simulink model "REDCS_Pipeline_IntermediateModel_FSU_29APR2022"  (R2022a)
settings: Solver=VariableStepAuto  StartTime=0.0  StopTime=3600  RelTol=1e-3
values from neighbouring files (symbols this model uses):
  Ac = (pi/4)*0.6096^2    (= 0.29186350796)    [REDCS_IntermediateModel_Parameters_29APR2022.m]
  B1 = 45    [REDCS_IntermediateModel_Parameters_29APR2022.m]
  CLOSED = 0    [REDCS_IntermediateModel_Parameters_29APR2022.m]
  EP020 = 21.9    [REDCS_IntermediateModel_Parameters_29APR2022.m]
  EP022 = 13.1    [REDCS_IntermediateModel_Parameters_29APR2022.m]
  EP024 = 54.2    [REDCS_IntermediateModel_Parameters_29APR2022.m]
  EP026 = 13.4    [REDCS_IntermediateModel_Parameters_29APR2022.m]
  EP028 = 0.5    [REDCS_IntermediateModel_Parameters_29APR2022.m]
  gamma = 1.2    [REDCS_IntermediateModel_Parameters_29APR2022.m]
  J = 5    [REDCS_IntermediateModel_Parameters_29APR2022.m]
  kf = 0.05    [REDCS_IntermediateModel_Parameters_29APR2022.m]
  Lc = 20    [REDCS_IntermediateModel_Parameters_29APR2022.m]
  OPEN = 1    [REDCS_IntermediateModel_Parameters_29APR2022.m]
  r1 = 0.05    [REDCS_IntermediateModel_Parameters_29APR2022.m]
  r2 = 0.325    [REDCS_IntermediateModel_Parameters_29APR2022.m]
  sigma = 0.90    (= 0.9)    [REDCS_IntermediateModel_Parameters_29APR2022.m]
  ValveThresh = 0.001    [REDCS_IntermediateModel_Parameters_29APR2022.m]
  ZR2000 = OPEN    (= 1)    [REDCS_IntermediateModel_Parameters_29APR2022.m]
  ZR2110 = CLOSED    (= 0)    [REDCS_IntermediateModel_Parameters_29APR2022.m]
  ZR2400 = OPEN    (= 1)    [REDCS_IntermediateModel_Parameters_29APR2022.m]
  ZR2401 = 100*OPEN    (= 100)    [REDCS_IntermediateModel_Parameters_29APR2022.m]
  ZR2510 = CLOSED    (= 0)    [REDCS_IntermediateModel_Parameters_29APR2022.m]
  ZR2600 = OPEN    (= 1)    [REDCS_IntermediateModel_Parameters_29APR2022.m]
  ZR2601 = 100*OPEN    (= 100)    [REDCS_IntermediateModel_Parameters_29APR2022.m]
  ZR2700 = OPEN    (= 1)    [REDCS_IntermediateModel_Parameters_29APR2022.m]
  ZR2701 = 100*OPEN    (= 100)    [REDCS_IntermediateModel_Parameters_29APR2022.m]
  ZR2800 = OPEN    (= 1)    [REDCS_IntermediateModel_Parameters_29APR2022.m]
  ZR2801 = 100*OPEN    (= 100)    [REDCS_IntermediateModel_Parameters_29APR2022.m]
  ZR2900 = OPEN    (= 1)    [REDCS_IntermediateModel_Parameters_29APR2022.m]
  ZR2901 = 100*OPEN    (= 100)    [REDCS_IntermediateModel_Parameters_29APR2022.m]
  ZR3900 = OPEN    (= 1)    [REDCS_IntermediateModel_Parameters_29APR2022.m]
  ZR4500 = OPEN    (= 1)    [REDCS_IntermediateModel_Parameters_29APR2022.m]
  ZR5600 = OPEN    (= 1)    [REDCS_IntermediateModel_Parameters_29APR2022.m]
  ZR7800 = CLOSED    (= 0)    [REDCS_IntermediateModel_Parameters_29APR2022.m]
undefined symbols (not defined in the file or in its folder): cotd, LEG_DEMAND_10A, LEG_DEMAND_3A, magnitude
libraries: fl_lib x170, nesl_utility x109, simulink x12, slpidlib x4
(part 4 of 4)

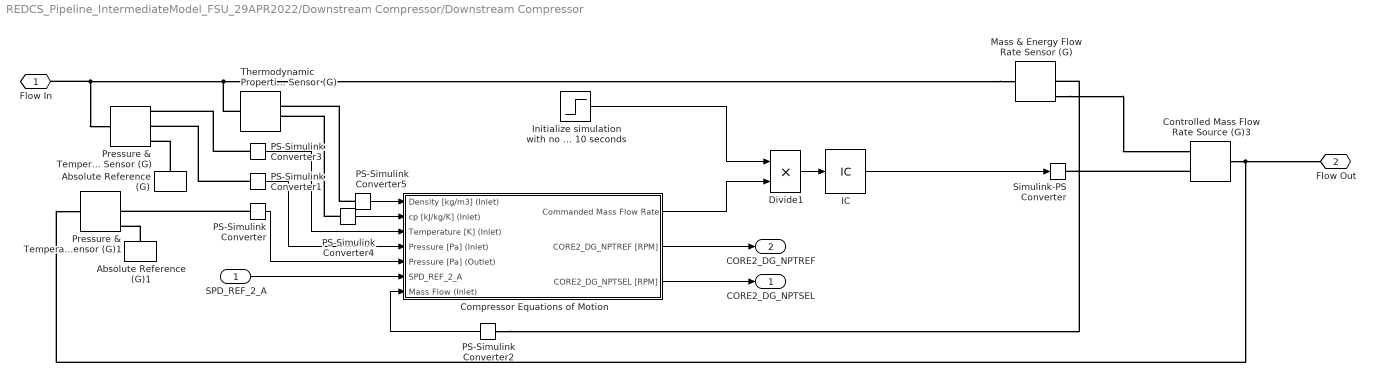
== system REDCS_Pipeline_IntermediateModel_FSU_29APR2022/Downstream Compressor/Downstream Compressor ==
  SPD_REF_2_A : Inport
  Absolute Reference (G) : fl_lib/Gas/Elements/Absolute Reference (G)
      settings: SourceProductBaseCode=PW,SS,VE  InternalSimscapePortConfiguration="{\"Bottom\":[],\"Left\":[{\"id\":\"A\",\"label\":\"\",\"type\":\"foundation.gas.gas\"}],\"Right\":[],\"Top\":[]}"
  Absolute Reference (G)1 : fl_lib/Gas/Elements/Absolute Reference (G)
      settings: SourceProductBaseCode=PW,SS,VE  InternalSimscapePortConfiguration="{\"Bottom\":[],\"Left\":[{\"id\":\"A\",\"label\":\"\",\"type\":\"foundation.gas.gas\"}],\"Right\":[],\"Top\":[]}"
  Compressor Equations of Motion : Subsystem
  Controlled Mass Flow Rate Source (G)3 : fl_lib/Gas/Sources/Controlled Mass Flow Rate Source (G)  power_spec=foundation.enum.power_spec.isentropic  area_A=(pi/4)*0.6096^2 m^2  area_B=(pi/4)*0.6096^2 m^2
      settings: SourceProductBaseCode=PW,SS,VE  InternalSimscapePortConfiguration="{\"Bottom\":[],\"Left\":[{\"id\":\"A\",\"label\":\"A\",\"type\":\"foundation.gas.gas\"},{\"id\":\"M\",\"label\":\"M\",\"type\":\"input\"}],\"Right\":[{\"id\":\"B\",\"label\":\"B\",\"type\":\"foundation.gas.gas\"}],\"Top\":[]}"
  Divide1 : Product  Inputs=**
  IC : InitialCondition  Value=0
  Initialize simulation with no flow from Compressor for first 10 seconds : Step  Time=10  SampleTime=0
  Mass & Energy Flow Rate Sensor (G) : fl_lib/Gas/Sensors/Mass & Energy Flow Rate Sensor (G)
      settings: SourceProductBaseCode=PW,SS,VE  InternalSimscapePortConfiguration="{\"Bottom\":[],\"Left\":[{\"id\":\"A\",\"label\":\"A\",\"type\":\"foundation.gas.gas\"}],\"Right\":[{\"id\":\"B\",\"label\":\"B\",\"type\":\"foundation.gas.gas\"},{\"id\":\"M\",\"label\":\"M\",\"type\":\"output\"},{\"id\":\"PHI\",\"label\":\"Phi\",\"type\":\"output\"}],\"Top\":[]}"
  PS-Simulink Converter{,1..5} (6 alike) : nesl_utility/PS-Simulink Converter  PhysicalDomain=network_engine_domain  SubClassName=ps_output  LeftPortType=input  RightPortType=output  PseudoPeriodic=off  Frequencies=[]  VectorFormat=1-D array  Unit=inherit  AffineConversion=off
      settings: SourceProductBaseCode=SS,PW,VE
  Pressure & Temperature Sensor (G) : fl_lib/Gas/Sensors/Pressure & Temperature Sensor (G)
      settings: SourceProductBaseCode=PW,SS,VE  InternalSimscapePortConfiguration="{\"Bottom\":[],\"Left\":[{\"id\":\"A\",\"label\":\"A\",\"type\":\"foundation.gas.gas\"}],\"Right\":[{\"id\":\"B\",\"label\":\"B\",\"type\":\"foundation.gas.gas\"},{\"id\":\"P\",\"label\":\"P\",\"type\":\"output\"},{\"id\":\"T\",\"label\":\"T\",\"type\":\"output\"}],\"Top\":[]}"
  Pressure & Temperature Sensor (G)1 : fl_lib/Gas/Sensors/Pressure & Temperature Sensor (G)
      settings: SourceProductBaseCode=PW,SS,VE  InternalSimscapePortConfiguration="{\"Bottom\":[],\"Left\":[{\"id\":\"A\",\"label\":\"A\",\"type\":\"foundation.gas.gas\"}],\"Right\":[{\"id\":\"B\",\"label\":\"B\",\"type\":\"foundation.gas.gas\"},{\"id\":\"P\",\"label\":\"P\",\"type\":\"output\"},{\"id\":\"T\",\"label\":\"T\",\"type\":\"output\"}],\"Top\":[]}"
  Simulink-PS Converter : nesl_utility/Simulink-PS Converter  PhysicalDomain=network_engine_domain  SubClassName=ps_input  LeftPortType=input  RightPortType=output  PseudoPeriodic=off  Frequencies=[]  NoiseDistribution=none  NoiseParameters=[]  Unit=1  AffineConversion=off  FilteringAndDerivatives=provide  SimscapeFilterOrder=1  InputFilterTimeConstant=0.001  UdotUserProvided=0
      settings: SourceProductBaseCode=SS,PW,VE
  Thermodynamic Properties Sensor (G) : fl_lib/Gas/Sensors/Thermodynamic Properties Sensor (G)  s_std=3.8635 kJ/kg/K  p_std=0.101325 MPa  T_std=293.15 K
      settings: SourceProductBaseCode=PW,SS,VE  InternalSimscapePortConfiguration="{\"Bottom\":[],\"Left\":[{\"id\":\"A\",\"label\":\"A\",\"type\":\"foundation.gas.gas\"}],\"Right\":[{\"id\":\"H\",\"label\":\"h\",\"type\":\"output\"},{\"id\":\"RHO\",\"label\":\"rho\",\"type\":\"output\"},{\"id\":\"CP\",\"label\":\"cp\",\"type\":\"output\"},{\"id\":\"S\",\"label\":\"s\",\"type\":\"output\"}],\"Top\":[]}"
  Flow In : PMIOPort  Side=Left
  Flow Out : PMIOPort  Port=2  Side=Right
  CORE2_DG_NPTSEL : Outport
  CORE2_DG_NPTREF : Outport  Port=2
  wires:
  SPD_REF_2_A/1 -> Compressor Equations of Motion/6(SPD_REF_2_A)
  PS-Simulink Converter1/1 -> Compressor Equations of Motion/4(Pressure [Pa] (Inlet))
  Compressor Equations of Motion/2(CORE2_DG_NPTREF [RPM]) -> CORE2_DG_NPTREF/1
  PS-Simulink Converter/1 -> Compressor Equations of Motion/5(Pressure [Pa] (Outlet))
  Compressor Equations of Motion/1(Commanded Mass Flow Rate) -> Divide1/2
  Initialize simulation with no flow from Compressor for first 10 seconds/1 -> Divide1/1
  Divide1/1 -> IC/1
  IC/1 -> Simulink-PS Converter/1
  PS-Simulink Converter2/1 -> Compressor Equations of Motion/7(Mass Flow (Inlet))
  PS-Simulink Converter3/1 -> Compressor Equations of Motion/3(Temperature [K] (Inlet))
  PS-Simulink Converter4/1 -> Compressor Equations of Motion/2(cp [kJ/kg/K] (Inlet))
  PS-Simulink Converter5/1 -> Compressor Equations of Motion/1(Density [kg/m3] (Inlet))
  Compressor Equations of Motion/3(CORE2_DG_NPTSEL [RPM]) -> CORE2_DG_NPTSEL/1
  connections:
  Mass & Energy Flow Rate Sensor (G)/LConn1 -- Pressure & Temperature Sensor (G)/LConn1 -- Flow In/RConn1 -- Thermodynamic Properties Sensor (G)/LConn1
  Controlled Mass Flow Rate Source (G)3/LConn2 -- Simulink-PS Converter/RConn1
  Controlled Mass Flow Rate Source (G)3/RConn1 -- Flow Out/RConn1 -- Pressure & Temperature Sensor (G)1/LConn1
  PS-Simulink Converter1/LConn1 -- Pressure & Temperature Sensor (G)/RConn2
  PS-Simulink Converter/LConn1 -- Pressure & Temperature Sensor (G)1/RConn2
  Absolute Reference (G)/LConn1 -- Pressure & Temperature Sensor (G)/RConn1
  Absolute Reference (G)1/LConn1 -- Pressure & Temperature Sensor (G)1/RConn1
  Mass & Energy Flow Rate Sensor (G)/RConn1 -- Controlled Mass Flow Rate Source (G)3/LConn1
  PS-Simulink Converter2/LConn1 -- Mass & Energy Flow Rate Sensor (G)/RConn2
  PS-Simulink Converter3/LConn1 -- Pressure & Temperature Sensor (G)/RConn3
  PS-Simulink Converter4/LConn1 -- Thermodynamic Properties Sensor (G)/RConn3
  PS-Simulink Converter5/LConn1 -- Thermodynamic Properties Sensor (G)/RConn2

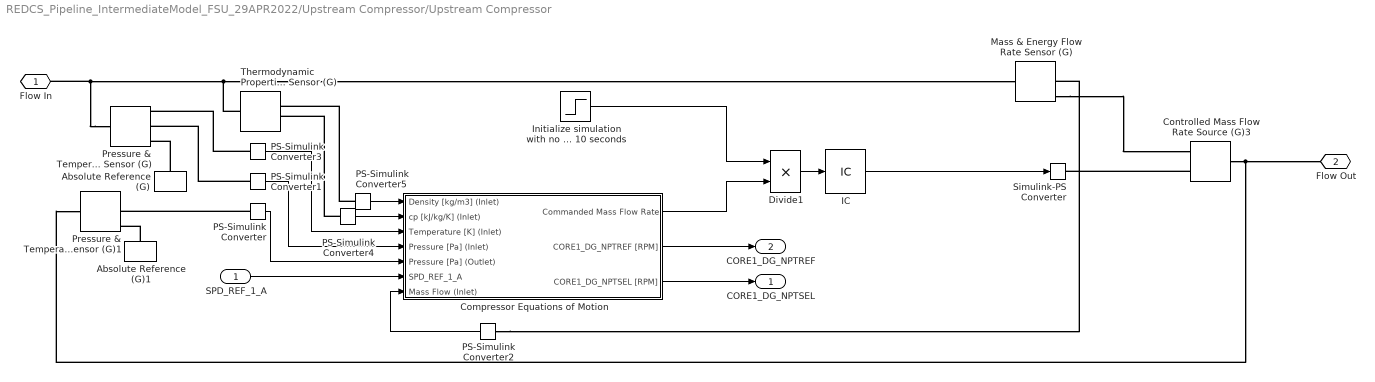
== system REDCS_Pipeline_IntermediateModel_FSU_29APR2022/Upstream Compressor/Upstream Compressor ==
  SPD_REF_1_A : Inport
  Absolute Reference (G) : fl_lib/Gas/Elements/Absolute Reference (G)
      settings: SourceProductBaseCode=PW,SS,VE  InternalSimscapePortConfiguration="{\"Bottom\":[],\"Left\":[{\"id\":\"A\",\"label\":\"\",\"type\":\"foundation.gas.gas\"}],\"Right\":[],\"Top\":[]}"
  Absolute Reference (G)1 : fl_lib/Gas/Elements/Absolute Reference (G)
      settings: SourceProductBaseCode=PW,SS,VE  InternalSimscapePortConfiguration="{\"Bottom\":[],\"Left\":[{\"id\":\"A\",\"label\":\"\",\"type\":\"foundation.gas.gas\"}],\"Right\":[],\"Top\":[]}"
  Compressor Equations of Motion : Subsystem
  Controlled Mass Flow Rate Source (G)3 : fl_lib/Gas/Sources/Controlled Mass Flow Rate Source (G)  power_spec=foundation.enum.power_spec.isentropic  area_A=(pi/4)*0.6096^2 m^2  area_B=(pi/4)*0.6096^2 m^2
      settings: SourceProductBaseCode=PW,SS,VE  InternalSimscapePortConfiguration="{\"Bottom\":[],\"Left\":[{\"id\":\"A\",\"label\":\"A\",\"type\":\"foundation.gas.gas\"},{\"id\":\"M\",\"label\":\"M\",\"type\":\"input\"}],\"Right\":[{\"id\":\"B\",\"label\":\"B\",\"type\":\"foundation.gas.gas\"}],\"Top\":[]}"
  Divide1 : Product  Inputs=**
  IC : InitialCondition  Value=0
  Initialize simulation with no flow from Compressor for first 10 seconds : Step  Time=10  SampleTime=0
  Mass & Energy Flow Rate Sensor (G) : fl_lib/Gas/Sensors/Mass & Energy Flow Rate Sensor (G)
      settings: SourceProductBaseCode=PW,SS,VE  InternalSimscapePortConfiguration="{\"Bottom\":[],\"Left\":[{\"id\":\"A\",\"label\":\"A\",\"type\":\"foundation.gas.gas\"}],\"Right\":[{\"id\":\"B\",\"label\":\"B\",\"type\":\"foundation.gas.gas\"},{\"id\":\"M\",\"label\":\"M\",\"type\":\"output\"},{\"id\":\"PHI\",\"label\":\"Phi\",\"type\":\"output\"}],\"Top\":[]}"
  PS-Simulink Converter{,1..5} (6 alike) : nesl_utility/PS-Simulink Converter  PhysicalDomain=network_engine_domain  SubClassName=ps_output  LeftPortType=input  RightPortType=output  PseudoPeriodic=off  Frequencies=[]  VectorFormat=1-D array  Unit=inherit  AffineConversion=off
      settings: SourceProductBaseCode=SS,PW,VE
  Pressure & Temperature Sensor (G) : fl_lib/Gas/Sensors/Pressure & Temperature Sensor (G)
      settings: SourceProductBaseCode=PW,SS,VE  InternalSimscapePortConfiguration="{\"Bottom\":[],\"Left\":[{\"id\":\"A\",\"label\":\"A\",\"type\":\"foundation.gas.gas\"}],\"Right\":[{\"id\":\"B\",\"label\":\"B\",\"type\":\"foundation.gas.gas\"},{\"id\":\"P\",\"label\":\"P\",\"type\":\"output\"},{\"id\":\"T\",\"label\":\"T\",\"type\":\"output\"}],\"Top\":[]}"
  Pressure & Temperature Sensor (G)1 : fl_lib/Gas/Sensors/Pressure & Temperature Sensor (G)
      settings: SourceProductBaseCode=PW,SS,VE  InternalSimscapePortConfiguration="{\"Bottom\":[],\"Left\":[{\"id\":\"A\",\"label\":\"A\",\"type\":\"foundation.gas.gas\"}],\"Right\":[{\"id\":\"B\",\"label\":\"B\",\"type\":\"foundation.gas.gas\"},{\"id\":\"P\",\"label\":\"P\",\"type\":\"output\"},{\"id\":\"T\",\"label\":\"T\",\"type\":\"output\"}],\"Top\":[]}"
  Simulink-PS Converter : nesl_utility/Simulink-PS Converter  PhysicalDomain=network_engine_domain  SubClassName=ps_input  LeftPortType=input  RightPortType=output  PseudoPeriodic=off  Frequencies=[]  NoiseDistribution=none  NoiseParameters=[]  Unit=1  AffineConversion=off  FilteringAndDerivatives=provide  SimscapeFilterOrder=1  InputFilterTimeConstant=0.001  UdotUserProvided=0
      settings: SourceProductBaseCode=SS,PW,VE
  Thermodynamic Properties Sensor (G) : fl_lib/Gas/Sensors/Thermodynamic Properties Sensor (G)  s_std=3.8635 kJ/kg/K  p_std=0.101325 MPa  T_std=293.15 K
      settings: SourceProductBaseCode=PW,SS,VE  InternalSimscapePortConfiguration="{\"Bottom\":[],\"Left\":[{\"id\":\"A\",\"label\":\"A\",\"type\":\"foundation.gas.gas\"}],\"Right\":[{\"id\":\"H\",\"label\":\"h\",\"type\":\"output\"},{\"id\":\"RHO\",\"label\":\"rho\",\"type\":\"output\"},{\"id\":\"CP\",\"label\":\"cp\",\"type\":\"output\"},{\"id\":\"S\",\"label\":\"s\",\"type\":\"output\"}],\"Top\":[]}"
  Flow In : PMIOPort  Side=Left
  Flow Out : PMIOPort  Port=2  Side=Right
  CORE1_DG_NPTSEL : Outport
  CORE1_DG_NPTREF : Outport  Port=2
  wires:
  SPD_REF_1_A/1 -> Compressor Equations of Motion/6(SPD_REF_1_A)
  PS-Simulink Converter1/1 -> Compressor Equations of Motion/4(Pressure [Pa] (Inlet))
  Compressor Equations of Motion/2(CORE1_DG_NPTREF [RPM]) -> CORE1_DG_NPTREF/1
  PS-Simulink Converter/1 -> Compressor Equations of Motion/5(Pressure [Pa] (Outlet))
  Compressor Equations of Motion/1(Commanded Mass Flow Rate) -> Divide1/2
  Initialize simulation with no flow from Compressor for first 10 seconds/1 -> Divide1/1
  Divide1/1 -> IC/1
  IC/1 -> Simulink-PS Converter/1
  PS-Simulink Converter2/1 -> Compressor Equations of Motion/7(Mass Flow (Inlet))
  PS-Simulink Converter3/1 -> Compressor Equations of Motion/3(Temperature [K] (Inlet))
  PS-Simulink Converter4/1 -> Compressor Equations of Motion/2(cp [kJ/kg/K] (Inlet))
  PS-Simulink Converter5/1 -> Compressor Equations of Motion/1(Density [kg/m3] (Inlet))
  Compressor Equations of Motion/3(CORE1_DG_NPTSEL [RPM]) -> CORE1_DG_NPTSEL/1
  connections:
  Pressure & Temperature Sensor (G)/LConn1 -- Thermodynamic Properties Sensor (G)/LConn1 -- Mass & Energy Flow Rate Sensor (G)/LConn1 -- Flow In/RConn1
  Controlled Mass Flow Rate Source (G)3/LConn2 -- Simulink-PS Converter/RConn1
  Controlled Mass Flow Rate Source (G)3/RConn1 -- Flow Out/RConn1 -- Pressure & Temperature Sensor (G)1/LConn1
  PS-Simulink Converter1/LConn1 -- Pressure & Temperature Sensor (G)/RConn2
  PS-Simulink Converter/LConn1 -- Pressure & Temperature Sensor (G)1/RConn2
  Absolute Reference (G)/LConn1 -- Pressure & Temperature Sensor (G)/RConn1
  Absolute Reference (G)1/LConn1 -- Pressure & Temperature Sensor (G)1/RConn1
  Mass & Energy Flow Rate Sensor (G)/RConn1 -- Controlled Mass Flow Rate Source (G)3/LConn1
  PS-Simulink Converter2/LConn1 -- Mass & Energy Flow Rate Sensor (G)/RConn2
  PS-Simulink Converter3/LConn1 -- Pressure & Temperature Sensor (G)/RConn3
  PS-Simulink Converter4/LConn1 -- Thermodynamic Properties Sensor (G)/RConn3
  PS-Simulink Converter5/LConn1 -- Thermodynamic Properties Sensor (G)/RConn2

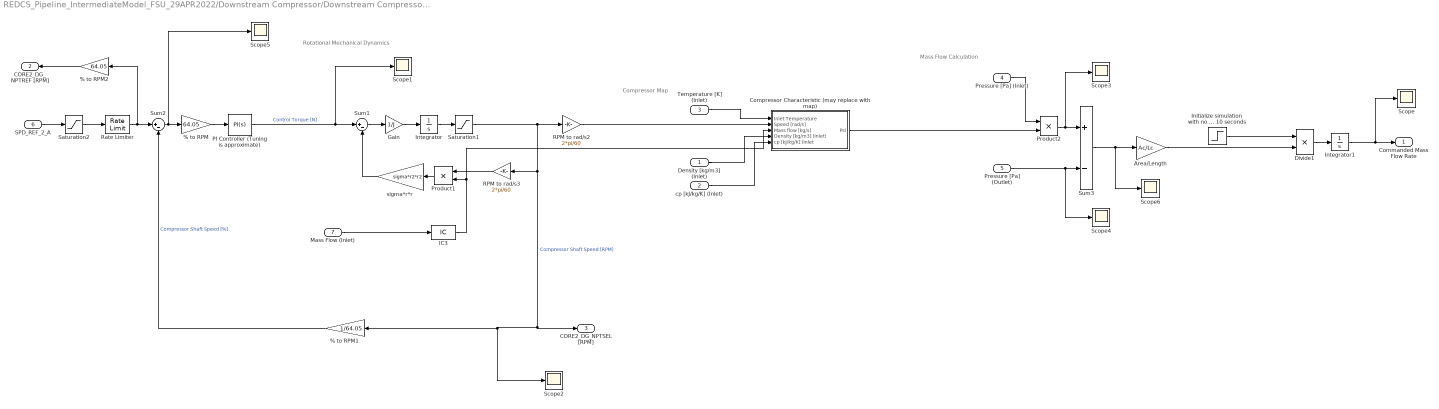
== system REDCS_Pipeline_IntermediateModel_FSU_29APR2022/Downstream Compressor/Downstream Compressor/Compressor Equations of Motion ==
  note: Rotational Mechanical Dynamics
  note: Compressor Map
  note: Mass Flow Calculation
  Density [kg/m3] (Inlet) : Inport
  cp [kJ/kg/K] (Inlet) : Inport  Port=2
  Temperature [K] (Inlet) : Inport  Port=3
  Pressure [Pa] (Inlet) : Inport  Port=4
  Pressure [Pa] (Outlet) : Inport  Port=5
  SPD_REF_2_A : Inport  Port=6
  Mass Flow (Inlet) : Inport  Port=7
  % to RPM : Gain  Gain=64.05
  % to RPM1 : Gain  Gain=1/64.05
  % to RPM2 : Gain  Gain=64.05
  Area/Length : Gain  Gain=Ac/Lc
  Compressor Characteristic (may replace with map) : Subsystem
  Divide1 : Product  Inputs=**
  Gain : Gain  Gain=1/J
  IC3 : InitialCondition  Value=0
  Initialize simulation with no flow from Compressor for first 10 seconds : Step  Time=10  SampleTime=0
  Integrator : Integrator
  Integrator1 : Integrator
  PI Controller (Tuning is approximate) : slpidlib/PID Controller  Controller=PI  Form=Parallel  TimeDomain=Continuous-time  UseExternalTs=off  SampleTime=-1  IntegratorMethod=Forward Euler  FilterMethod=Forward Euler  ControllerParametersSource=internal  P=10  I=1  UseKiTs=off  D=0  N=100  UseFilter=on  TunerSelectOption=Transfer Function Based (PID Tuner App)  InitialConditionSource=internal  InitialConditionForIntegrator=0  InitialConditionForFilter=0  DifferentiatorICPrevScaledInput=0  ExternalReset=none  TrackingMode=off  Kt=1  LimitOutput=off  SatLimitsSource=internal  UpperSaturationLimit=inf  LowerSaturationLimit=-inf  LinearizeAsGain=on  AntiWindupMode=none  Kb=1  POutMin=[]  POutMax=[]  IOutMin=[]  IOutMax=[]  DOutMin=[]  DOutMax=[]  NOutMin=[]  NOutMax=[]  SumOutMin=[]  SumOutMax=[]  SaturationOutMin=[]  SaturationOutMax=[]  PParamMin=[]  PParamMax=[]  IParamMin=[]  IParamMax=[]  DParamMin=[]  DParamMax=[]  NParamMin=[]  NParamMax=[]  KbParamMin=[]  KbParamMax=[]  KtParamMin=[]  KtParamMax=[]  KbOutMin=[]  KbOutMax=[]  KtOutMin=[]  KtOutMax=[]  IntegratorOutMin=[]  IntegratorOutMax=[]  FilterOutMin=[]  FilterOutMax=[]  SumI1OutMin=[]  SumI1OutMax=[]  SumI2OutMin=[]  SumI2OutMax=[]  SumI3OutMin=[]  SumI3OutMax=[]  SumI4OutMin=[]  SumI4OutMax=[]  SumDOutMin=[]  SumDOutMax=[]  DifferentiatorOutMin=[]  DifferentiatorOutMax=[]  FilterDiffOutCoefMin=[]  FilterDiffOutCoefMax=[]  ReciprocalOutMin=[]  ReciprocalOutMax=[]  SumDenOutMin=[]  SumDenOutMax=[]  SumNumOutMin=[]  SumNumOutMax=[]  DivideOutMin=[]  DivideOutMax=[]  UdiffTsProdOutMin=[]  UdiffTsProdOutMax=[]  NTsProdOutMin=[]  NTsProdOutMax=[]  UintegralTsProdOutMin=[]  UintegralTsProdOutMax=[]  UngainTsProdOutMin=[]  UngainTsProdOutMax=[]  IntegratorContinuousStateAttributes=''  IntegratorStateMustResolveToSignalObject=off  IntegratorRTWStateStorageClass=Auto  FilterContinuousStateAttributes=''  FilterStateMustResolveToSignalObject=off  FilterRTWStateStorageClass=Auto  ParallelPVariant=InternalParameters  IdealPVariant=Disabled  IVariant=InternalParameters  DVariant=Disabled  IntegratorVariant=Continuous  SatVariant=Disabled  AWVariant=Passthrough  PCopyVariant=Disabled  TRVariant=Disabled  FdbkBlocksVariant=Forward  IdealPFdbkVariant=Disabled  SatFdbkVariant=Disabled  DerivativeFilterVariant=Disabled  NVariant=Disabled  NCopyVariant=Disabled_SignalSpec  FilterICVariant=Disabled  IntegratorICVariant=InternalICs  ExternalResetVariant=Disabled  TRSumVariant=Passthrough  SumFdbkVariant=Disabled  SumVariant=Sum_PI  TsampFilterVariant=InternalTs  TsampNgainVariant=Passthrough  TsampIntegralVariant=Passthrough  ExternalSaturationOutDataTypeStr=Inherit: Same as second input  aMode=0
  Product1 : Product
  Product2 : Product
  RPM to rad/s2 : Gain  Gain=2*pi/60
  RPM to rad/s3 : Gain  Gain=2*pi/60
  Rate Limiter : RateLimiter  RisingSlewLimit=0.035  FallingSlewLimit=-0.035  SampleTimeMode=inherited  InitialCondition=77
  Saturation1 : Saturate  UpperLimit=6405  LowerLimit=0
  Saturation2 : Saturate  UpperLimit=100  LowerLimit=0
  Scope{,1..6} (7 alike) : Scope
  Sum1 : Sum  Inputs=|+-
  Sum2 : Sum  Inputs=|+-
  Sum3 : Sum  Inputs=+-
  sigma*r*r : Gain  Gain=sigma*r2*r2
  Commanded Mass Flow Rate : Outport
  CORE2_DG_NPTREF [RPM] : Outport  Port=2
  CORE2_DG_NPTSEL [RPM] : Outport  Port=3
  wires:
  SPD_REF_2_A/1 -> Saturation2/1
  Saturation2/1 -> Rate Limiter/1
  Rate Limiter/1 -> % to RPM2/1, Sum2/1
  Mass Flow (Inlet)/1 -> IC3/1
  Sum2/1 -> Scope5/1, % to RPM/1
  PI Controller (Tuning is approximate)/1 -> Scope1/1, Sum1/1  "Control Torque [N]"
  Product1/1 -> sigma*r*r/1
  IC3/1 -> Product1/2, Compressor Characteristic (may replace with map)/3(Mass flow [kg/s])
  Sum1/1 -> Gain/1
  sigma*r*r/1 -> Sum1/2
  Gain/1 -> Integrator/1
  Compressor Characteristic (may replace with map)/1(Psi) -> Product2/2
  Pressure [Pa] (Inlet)/1 -> Product2/1
  Product2/1 -> Scope3/1, Sum3/1
  Pressure [Pa] (Outlet)/1 -> Scope4/1, Sum3/2
  Area/Length/1 -> Divide1/2
  Integrator/1 -> Saturation1/1
  % to RPM/1 -> PI Controller (Tuning is approximate)/1
  Saturation1/1 -> RPM to rad/s2/1, Scope2/1, % to RPM1/1, CORE2_DG_NPTSEL [RPM]/1, RPM to rad/s3/1  "Compressor Shaft Speed [RPM]"
  RPM to rad/s3/1 -> Product1/1
  Density [kg/m3] (Inlet)/1 -> Compressor Characteristic (may replace with map)/4(Density [kg/m3] (Inlet))
  cp [kJ/kg/K] (Inlet)/1 -> Compressor Characteristic (may replace with map)/5(cp [kJ/kg/K] (Inlet)
  Temperature [K] (Inlet)/1 -> Compressor Characteristic (may replace with map)/1(Inlet Temperature)
  RPM to rad/s2/1 -> Compressor Characteristic (may replace with map)/2(Speed [rad/s])
  Integrator1/1 -> Scope/1, Commanded Mass Flow Rate/1
  % to RPM1/1 -> Sum2/2  "Compressor Shaft Speed [%]"
  Initialize simulation with no flow from Compressor for first 10 seconds/1 -> Divide1/1
  Divide1/1 -> Integrator1/1
  Sum3/1 -> Scope6/1, Area/Length/1
  % to RPM2/1 -> CORE2_DG_NPTREF [RPM]/1

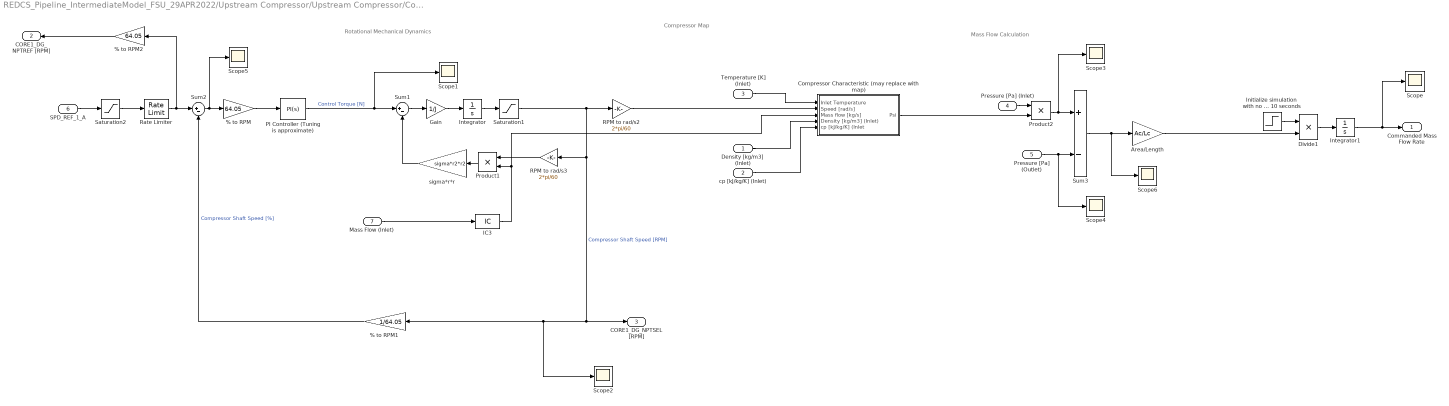
== system REDCS_Pipeline_IntermediateModel_FSU_29APR2022/Upstream Compressor/Upstream Compressor/Compressor Equations of Motion ==
  note: Rotational Mechanical Dynamics
  note: Compressor Map
  note: Mass Flow Calculation
  Density [kg/m3] (Inlet) : Inport
  cp [kJ/kg/K] (Inlet) : Inport  Port=2
  Temperature [K] (Inlet) : Inport  Port=3
  Pressure [Pa] (Inlet) : Inport  Port=4
  Pressure [Pa] (Outlet) : Inport  Port=5
  SPD_REF_1_A : Inport  Port=6
  Mass Flow (Inlet) : Inport  Port=7
  % to RPM : Gain  Gain=64.05
  % to RPM1 : Gain  Gain=1/64.05
  % to RPM2 : Gain  Gain=64.05
  Area/Length : Gain  Gain=Ac/Lc
  Compressor Characteristic (may replace with map) : Subsystem
  Divide1 : Product  Inputs=**
  Gain : Gain  Gain=1/J
  IC3 : InitialCondition  Value=0
  Initialize simulation with no flow from Compressor for first 10 seconds : Step  Time=10  SampleTime=0
  Integrator : Integrator
  Integrator1 : Integrator
  PI Controller (Tuning is approximate) : slpidlib/PID Controller  Controller=PI  Form=Parallel  TimeDomain=Continuous-time  UseExternalTs=off  SampleTime=-1  IntegratorMethod=Forward Euler  FilterMethod=Forward Euler  ControllerParametersSource=internal  P=10  I=1  UseKiTs=off  D=0  N=100  UseFilter=on  TunerSelectOption=Transfer Function Based (PID Tuner App)  InitialConditionSource=internal  InitialConditionForIntegrator=0  InitialConditionForFilter=0  DifferentiatorICPrevScaledInput=0  ExternalReset=none  TrackingMode=off  Kt=1  LimitOutput=off  SatLimitsSource=internal  UpperSaturationLimit=inf  LowerSaturationLimit=-inf  LinearizeAsGain=on  AntiWindupMode=none  Kb=1  POutMin=[]  POutMax=[]  IOutMin=[]  IOutMax=[]  DOutMin=[]  DOutMax=[]  NOutMin=[]  NOutMax=[]  SumOutMin=[]  SumOutMax=[]  SaturationOutMin=[]  SaturationOutMax=[]  PParamMin=[]  PParamMax=[]  IParamMin=[]  IParamMax=[]  DParamMin=[]  DParamMax=[]  NParamMin=[]  NParamMax=[]  KbParamMin=[]  KbParamMax=[]  KtParamMin=[]  KtParamMax=[]  KbOutMin=[]  KbOutMax=[]  KtOutMin=[]  KtOutMax=[]  IntegratorOutMin=[]  IntegratorOutMax=[]  FilterOutMin=[]  FilterOutMax=[]  SumI1OutMin=[]  SumI1OutMax=[]  SumI2OutMin=[]  SumI2OutMax=[]  SumI3OutMin=[]  SumI3OutMax=[]  SumI4OutMin=[]  SumI4OutMax=[]  SumDOutMin=[]  SumDOutMax=[]  DifferentiatorOutMin=[]  DifferentiatorOutMax=[]  FilterDiffOutCoefMin=[]  FilterDiffOutCoefMax=[]  ReciprocalOutMin=[]  ReciprocalOutMax=[]  SumDenOutMin=[]  SumDenOutMax=[]  SumNumOutMin=[]  SumNumOutMax=[]  DivideOutMin=[]  DivideOutMax=[]  UdiffTsProdOutMin=[]  UdiffTsProdOutMax=[]  NTsProdOutMin=[]  NTsProdOutMax=[]  UintegralTsProdOutMin=[]  UintegralTsProdOutMax=[]  UngainTsProdOutMin=[]  UngainTsProdOutMax=[]  IntegratorContinuousStateAttributes=''  IntegratorStateMustResolveToSignalObject=off  IntegratorRTWStateStorageClass=Auto  FilterContinuousStateAttributes=''  FilterStateMustResolveToSignalObject=off  FilterRTWStateStorageClass=Auto  ParallelPVariant=InternalParameters  IdealPVariant=Disabled  IVariant=InternalParameters  DVariant=Disabled  IntegratorVariant=Continuous  SatVariant=Disabled  AWVariant=Passthrough  PCopyVariant=Disabled  TRVariant=Disabled  FdbkBlocksVariant=Forward  IdealPFdbkVariant=Disabled  SatFdbkVariant=Disabled  DerivativeFilterVariant=Disabled  NVariant=Disabled  NCopyVariant=Disabled_SignalSpec  FilterICVariant=Disabled  IntegratorICVariant=InternalICs  ExternalResetVariant=Disabled  TRSumVariant=Passthrough  SumFdbkVariant=Disabled  SumVariant=Sum_PI  TsampFilterVariant=InternalTs  TsampNgainVariant=Passthrough  TsampIntegralVariant=Passthrough  ExternalSaturationOutDataTypeStr=Inherit: Same as second input  aMode=0
  Product1 : Product
  Product2 : Product
  RPM to rad/s2 : Gain  Gain=2*pi/60
  RPM to rad/s3 : Gain  Gain=2*pi/60
  Rate Limiter : RateLimiter  RisingSlewLimit=0.035  FallingSlewLimit=-0.035  SampleTimeMode=inherited  InitialCondition=77
  Saturation1 : Saturate  UpperLimit=6405  LowerLimit=0
  Saturation2 : Saturate  UpperLimit=100  LowerLimit=0
  Scope{,1..6} (7 alike) : Scope
  Sum1 : Sum  Inputs=|+-
  Sum2 : Sum  Inputs=|+-
  Sum3 : Sum  Inputs=+-
  sigma*r*r : Gain  Gain=sigma*r2*r2
  Commanded Mass Flow Rate : Outport
  CORE1_DG_NPTREF [RPM] : Outport  Port=2
  CORE1_DG_NPTSEL [RPM] : Outport  Port=3
  wires:
  SPD_REF_1_A/1 -> Saturation2/1
  Saturation2/1 -> Rate Limiter/1
  Rate Limiter/1 -> % to RPM2/1, Sum2/1
  Mass Flow (Inlet)/1 -> IC3/1
  Sum2/1 -> Scope5/1, % to RPM/1
  PI Controller (Tuning is approximate)/1 -> Scope1/1, Sum1/1  "Control Torque [N]"
  Product1/1 -> sigma*r*r/1
  IC3/1 -> Product1/2, Compressor Characteristic (may replace with map)/3(Mass flow [kg/s])
  Sum1/1 -> Gain/1
  sigma*r*r/1 -> Sum1/2
  Gain/1 -> Integrator/1
  Compressor Characteristic (may replace with map)/1(Psi) -> Product2/2
  Pressure [Pa] (Inlet)/1 -> Product2/1
  Product2/1 -> Scope3/1, Sum3/1
  Pressure [Pa] (Outlet)/1 -> Scope4/1, Sum3/2
  Area/Length/1 -> Divide1/2
  Integrator/1 -> Saturation1/1
  % to RPM/1 -> PI Controller (Tuning is approximate)/1
  Saturation1/1 -> RPM to rad/s2/1, Scope2/1, % to RPM1/1, CORE1_DG_NPTSEL [RPM]/1, RPM to rad/s3/1  "Compressor Shaft Speed [RPM]"
  RPM to rad/s3/1 -> Product1/1
  Density [kg/m3] (Inlet)/1 -> Compressor Characteristic (may replace with map)/4(Density [kg/m3] (Inlet))
  cp [kJ/kg/K] (Inlet)/1 -> Compressor Characteristic (may replace with map)/5(cp [kJ/kg/K] (Inlet)
  Temperature [K] (Inlet)/1 -> Compressor Characteristic (may replace with map)/1(Inlet Temperature)
  RPM to rad/s2/1 -> Compressor Characteristic (may replace with map)/2(Speed [rad/s])
  Integrator1/1 -> Scope/1, Commanded Mass Flow Rate/1
  % to RPM1/1 -> Sum2/2  "Compressor Shaft Speed [%]"
  Initialize simulation with no flow from Compressor for first 10 seconds/1 -> Divide1/1
  Divide1/1 -> Integrator1/1
  Sum3/1 -> Scope6/1, Area/Length/1
  % to RPM2/1 -> CORE1_DG_NPTREF [RPM]/1

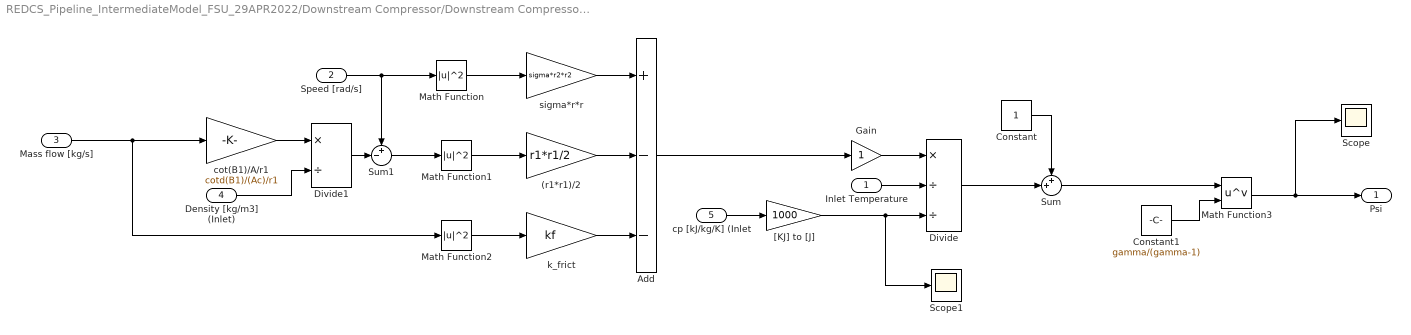
== system REDCS_Pipeline_IntermediateModel_FSU_29APR2022/Downstream Compressor/Downstream Compressor/Compressor Equations of Motion/Compressor Characteristic (may replace with map) ==
  Inlet Temperature : Inport
  Speed [rad/s] : Inport  Port=2
  Mass flow [kg/s] : Inport  Port=3
  Density [kg/m3] (Inlet) : Inport  Port=4
  cp [kJ/kg/K] (Inlet : Inport  Port=5
  (r1*r1)/2 : Gain  Gain=r1*r1/2
  Add : Sum  Inputs=+--
  Constant : Constant
  Constant1 : Constant  Value=gamma/(gamma-1)
  Divide : Product  Inputs=*//
  Divide1 : Product  Inputs=*/
  Gain : Gain
  Math Function : Math  Operator=magnitude^2
  Math Function1 : Math  Operator=magnitude^2
  Math Function2 : Math  Operator=magnitude^2
  Math Function3 : Math  Operator=pow
  Scope : Scope
  Scope1 : Scope
  Sum : Sum  Inputs=++|
  Sum1 : Sum  Inputs=+-|
  "[KJ] to [J]" : Gain  Gain=1000
  cot(B1)/A/r1 : Gain  Gain=cotd(B1)/(Ac)/r1
  k_frict : Gain  Gain=kf
  sigma*r*r : Gain  Gain=sigma*r2*r2
  Psi : Outport
  wires:
  Sum/1 -> Math Function3/1
  Constant/1 -> Sum/1
  Gain/1 -> Divide/1
  Divide/1 -> Sum/2
  Inlet Temperature/1 -> Divide/2
  Add/1 -> Gain/1
  Speed [rad/s]/1 -> Math Function/1, Sum1/1
  Math Function/1 -> sigma*r*r/1
  sigma*r*r/1 -> Add/1
  cp [kJ/kg/K] (Inlet/1 -> "[KJ] to [J]"/1
  "[KJ] to [J]"/1 -> Scope1/1, Divide/3
  (r1*r1)/2/1 -> Add/2
  cot(B1)/A/r1/1 -> Divide1/1
  Density [kg/m3] (Inlet)/1 -> Divide1/2
  Divide1/1 -> Sum1/2
  Math Function1/1 -> (r1*r1)/2/1
  Sum1/1 -> Math Function1/1
  Mass flow [kg/s]/1 -> Math Function2/1, cot(B1)/A/r1/1
  k_frict/1 -> Add/3
  Math Function2/1 -> k_frict/1
  Math Function3/1 -> Scope/1, Psi/1
  Constant1/1 -> Math Function3/2

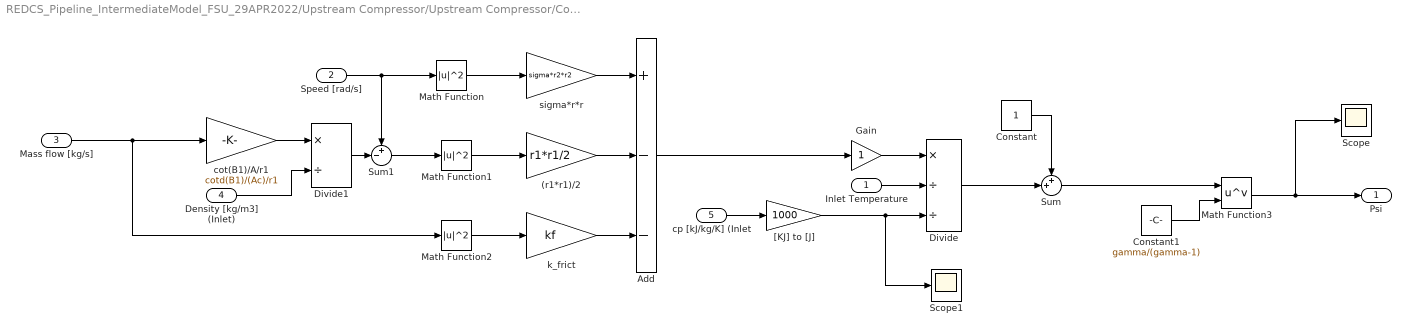
== system REDCS_Pipeline_IntermediateModel_FSU_29APR2022/Upstream Compressor/Upstream Compressor/Compressor Equations of Motion/Compressor Characteristic (may replace with map) ==
  Inlet Temperature : Inport
  Speed [rad/s] : Inport  Port=2
  Mass flow [kg/s] : Inport  Port=3
  Density [kg/m3] (Inlet) : Inport  Port=4
  cp [kJ/kg/K] (Inlet : Inport  Port=5
  (r1*r1)/2 : Gain  Gain=r1*r1/2
  Add : Sum  Inputs=+--
  Constant : Constant
  Constant1 : Constant  Value=gamma/(gamma-1)
  Divide : Product  Inputs=*//
  Divide1 : Product  Inputs=*/
  Gain : Gain
  Math Function : Math  Operator=magnitude^2
  Math Function1 : Math  Operator=magnitude^2
  Math Function2 : Math  Operator=magnitude^2
  Math Function3 : Math  Operator=pow
  Scope : Scope
  Scope1 : Scope
  Sum : Sum  Inputs=++|
  Sum1 : Sum  Inputs=+-|
  "[KJ] to [J]" : Gain  Gain=1000
  cot(B1)/A/r1 : Gain  Gain=cotd(B1)/(Ac)/r1
  k_frict : Gain  Gain=kf
  sigma*r*r : Gain  Gain=sigma*r2*r2
  Psi : Outport
  wires:
  Sum/1 -> Math Function3/1
  Constant/1 -> Sum/1
  Gain/1 -> Divide/1
  Divide/1 -> Sum/2
  Inlet Temperature/1 -> Divide/2
  Add/1 -> Gain/1
  Speed [rad/s]/1 -> Math Function/1, Sum1/1
  Math Function/1 -> sigma*r*r/1
  sigma*r*r/1 -> Add/1
  cp [kJ/kg/K] (Inlet/1 -> "[KJ] to [J]"/1
  "[KJ] to [J]"/1 -> Scope1/1, Divide/3
  (r1*r1)/2/1 -> Add/2
  cot(B1)/A/r1/1 -> Divide1/1
  Density [kg/m3] (Inlet)/1 -> Divide1/2
  Divide1/1 -> Sum1/2
  Math Function1/1 -> (r1*r1)/2/1
  Sum1/1 -> Math Function1/1
  Mass flow [kg/s]/1 -> Math Function2/1, cot(B1)/A/r1/1
  k_frict/1 -> Add/3
  Math Function2/1 -> k_frict/1
  Math Function3/1 -> Scope/1, Psi/1
  Constant1/1 -> Math Function3/2
